simulink model "KinematicModel1"  (R2024a)
settings: Solver=FixedStepAuto  StartTime=0.0  StopTime=10.0  RelTol=1e-3
settings Model: Creator=levirogalla  LastModifiedBy=levirogalla

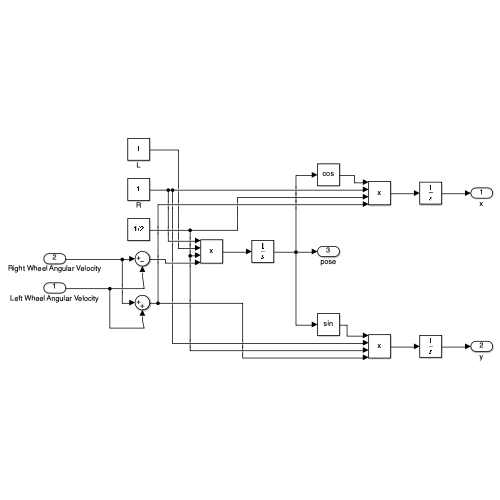
[thumbnail: Simulink's stored preview of the top-level diagram]
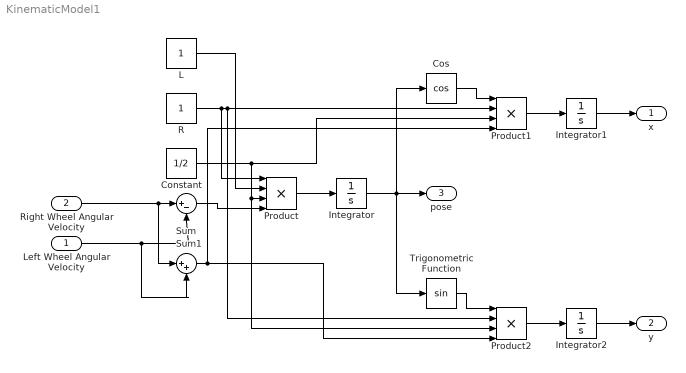
== system KinematicModel1 ==
  Left Wheel Angular Velocity : Inport
  Right Wheel Angular Velocity : Inport  Port=2
  Constant : Constant  Value=1/2
  Cos : Trigonometry  Operator=cos
  Integrator : Integrator
  Integrator1 : Integrator
  Integrator2 : Integrator
  L : Constant  Description=Centriod to wheel length
  Product : Product  Inputs=4
  Product1 : Product  Inputs=4
  Product2 : Product  Inputs=4
  R : Constant  Description=The radius of the wheels
  Sum : Sum  Inputs=|+-
  Sum1 : Sum  Inputs=|++
  Trigonometric Function : Trigonometry
  x : Outport
  y : Outport  Port=2
  pose : Outport  Port=3
  wires:
  Integrator1/1 -> x/1
  Integrator2/1 -> y/1
  Product2/1 -> Integrator2/1
  Product1/1 -> Integrator1/1
  Left Wheel Angular Velocity/1 -> Sum/2, Sum1/2
  Trigonometric Function/1 -> Product2/1
  Sum1/1 -> Product1/4, Product2/4
  Sum/1 -> Product/4
  R/1 -> Product2/2, Product1/2, Product/1
  L/1 -> Product/2
  Integrator/1 -> pose/1, Cos/1, Trigonometric Function/1
  Product/1 -> Integrator/1
  Cos/1 -> Product1/1
  Constant/1 -> Product/3, Product2/3, Product1/3
  Right Wheel Angular Velocity/1 -> Sum1/1, Sum/1
